simulink model "Room"  (R2016b)
settings: Solver=FixedStepDiscrete  StartTime=0.0  StopTime=10.0  FixedStep=.0001  RelTol=1e-3
settings Model: Creator=3essawy  LastModifiedBy=3essawy
settings OptimizationCC: DefaultParameterBehavior=Inlined
settings DebuggingCC: ParameterTunabilityLossMsg=error
settings RTWCC: SystemTargetFile=ert.tlc  GenCodeOnly=on  TemplateMakefile=ert_default_tmf  Description=Embedded Coder  GenerateReport=on  IncludeHyperlinkInReport=on  LaunchReport=on  GenerateTraceInfo=on  GenerateTraceReport=on  GenerateTraceReportSl=on  GenerateTraceReportSf=on  GenerateTraceReportEml=on
settings CodeAppCC: ForceParamTrailComments=on  IgnoreCustomStorageClasses=off  OperatorAnnotations=on  SimulinkDataObjDesc=on  SFDataObjDesc=on  MATLABFcnDesc=on  InsertBlockDesc=on  MATLABSourceComments=on
settings ERTTargetCC: TargetLangStandard=C99 (ISO)  GenerateSampleERTMain=on  InlinedParameterPlacement=NonHierarchical  ERTCustomFileTemplate=example_file_process.tlc  EnableUserReplacementTypes=on

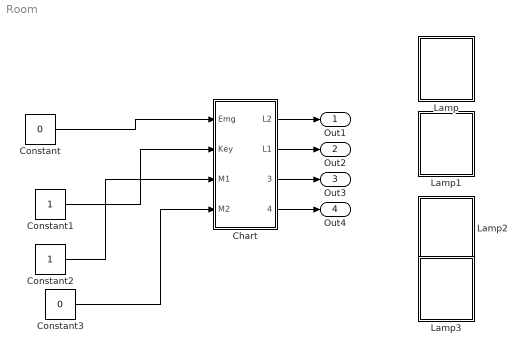
== system Room ==
  Chart : Stateflow chart  TreatAsAtomicUnit=on
  Constant : Constant  Value=0
  Constant1 : Constant
  Constant2 : Constant
  Constant3 : Constant  Value=0
  Lamp : Subsystem  DialogController=hmiCreateDDGDialog  IsWebBlock=on  mask(MWDashboardBlock){webBlockId=adf13d67-74a8-4b5f-91b1-061ae6b7b762, webBlockType=lamp, ShowInLibBrowser=on, ShowInitialText=on, HMISrcModelName=Room}
      mask prompts: webBlockType "WebBlock Type"; HMISrcModelName "Source Model"
      mask help: SimulinkHMI:dialogs:LampDialogDesc
      mask Help: helpview([docroot '/mapfiles/simulink.map'], 'hmi_lamp')
      mask Display:
      | if strcmp(get_param(bdroot(gcb),'BlockDiagramType'), 'library')
      |     image([(matlabroot) '/toolbox/simulink/hmi/icons/Lamp.png']);
      | end
  Lamp1 : Subsystem  DialogController=hmiCreateDDGDialog  IsWebBlock=on  mask(MWDashboardBlock){webBlockId=1f721917-04ac-4bba-95fc-ec4be05f69ce, webBlockType=lamp, ShowInLibBrowser=on, ShowInitialText=on, HMISrcModelName=Room}
      mask prompts: webBlockType "WebBlock Type"; HMISrcModelName "Source Model"
      mask help: SimulinkHMI:dialogs:LampDialogDesc
      mask Help: helpview([docroot '/mapfiles/simulink.map'], 'hmi_lamp')
      mask Display:
      | if strcmp(get_param(bdroot(gcb),'BlockDiagramType'), 'library')
      |     image([(matlabroot) '/toolbox/simulink/hmi/icons/Lamp.png']);
      | end
  Lamp2 : Subsystem  DialogController=hmiCreateDDGDialog  IsWebBlock=on  mask(MWDashboardBlock){webBlockId=013104e0-6487-4568-8424-da7791aa4bbe, webBlockType=lamp, ShowInLibBrowser=on, ShowInitialText=on, HMISrcModelName=Room}
      mask prompts: webBlockType "WebBlock Type"; HMISrcModelName "Source Model"
      mask help: SimulinkHMI:dialogs:LampDialogDesc
      mask Help: helpview([docroot '/mapfiles/simulink.map'], 'hmi_lamp')
      mask Display:
      | if strcmp(get_param(bdroot(gcb),'BlockDiagramType'), 'library')
      |     image([(matlabroot) '/toolbox/simulink/hmi/icons/Lamp.png']);
      | end
  Lamp3 : Subsystem  DialogController=hmiCreateDDGDialog  IsWebBlock=on  mask(MWDashboardBlock){webBlockId=04b49fa6-c082-4da2-bee2-49062ed6e447, webBlockType=lamp, ShowInLibBrowser=on, ShowInitialText=on, HMISrcModelName=Room}
      mask prompts: webBlockType "WebBlock Type"; HMISrcModelName "Source Model"
      mask help: SimulinkHMI:dialogs:LampDialogDesc
      mask Help: helpview([docroot '/mapfiles/simulink.map'], 'hmi_lamp')
      mask Display:
      | if strcmp(get_param(bdroot(gcb),'BlockDiagramType'), 'library')
      |     image([(matlabroot) '/toolbox/simulink/hmi/icons/Lamp.png']);
      | end
  Out1 : Outport
  Out2 : Outport  Port=2
  Out3 : Outport  Port=3
  Out4 : Outport  Port=4
  wires:
  Chart/1(L2) -> Out1/1
  Chart/2(L1) -> Out2/1
  Chart/3(GateLock) -> Out3/1
  Chart/4(Vacum) -> Out4/1
  Constant/1 -> Chart/1(Emg)
  Constant1/1 -> Chart/2(Key)
  Constant2/1 -> Chart/3(M1)
  Constant3/1 -> Chart/4(M2)

== system Room/Lamp ==

== system Room/Lamp1 ==

== system Room/Lamp2 ==

== system Room/Lamp3 ==

== stateflow chart Room/Chart ==
  state Inavalid
  state Valid
    entry:
  state Vac
    entry:
    Vacum=1;
    GateLock=1;
  state R1
    entry:
    L1=1;
    exit:
    L1=0;
  state R2
    entry:
    L2=1;
    exit:
    L2=0;
  state Emg
    entry:
    L1=1;
    L2=1;
  Vac -> Valid
  (default) -> Valid
  Valid -> R1 [order 2] : [M1==1]
  Valid -> Inavalid [order 1] : [Key==0]
  Inavalid -> Valid : [Key==1]
  R1 -> Valid [order 1] : [M1==0]
  R2 -> Valid [order 1] : [M2==0]
  Valid -> R2 [order 3] : [M2==1]
  Valid -> Emg [order 4] : [Emg==1]
  Emg -> Vac : after(5,sec)
  R1 -> R2 [order 2] : [M1==0]
  R2 -> R1 [order 2] : [M2==0]
  data: Emg input; Key input; L2 output; L1 output; GateLock output; Vacum output; M1 input; M2 input
